simulink model "hw4q1a"  (R2019b)
settings: Solver=FixedStepAuto  StartTime=0.0  StopTime=20  FixedStep=0.01  RelTol=1e-3
libraries: slident x2
settings Model: Creator=axs2437  LastModifiedBy=axs2437
settings DataIOCC: ReturnWorkspaceOutputs=off

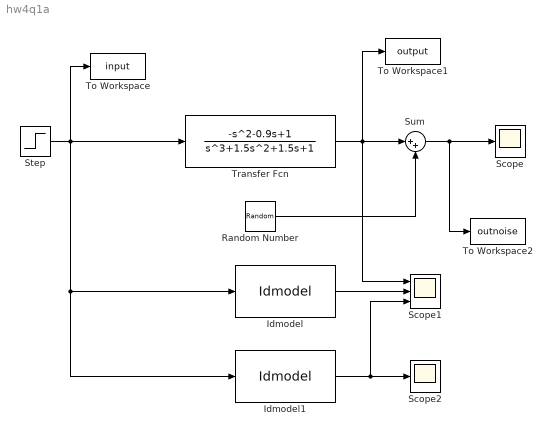
== system hw4q1a ==
  Idmodel : slident/Models/Idmodel  sys=arx321  IC=0  noi=off  seed=[]
      settings: SourceProductName=System Identification Toolbox  SourceProductBaseCode=ID
  Idmodel1 : slident/Models/Idmodel  sys=arx541  IC=0  noi=off  seed=[]
      settings: SourceProductName=System Identification Toolbox  SourceProductBaseCode=ID
  Random Number : RandomNumber  Variance=0.001  SampleTime=0.01
  Scope : Scope
  Scope1 : Scope  NumInputPorts=3
  Scope2 : Scope
  Step : Step  SampleTime=0.01
  Sum : Sum  Inputs=|++
  To Workspace : ToWorkspace  VariableName=input  SampleTime=-1
  To Workspace1 : ToWorkspace  VariableName=output  SampleTime=-1
  To Workspace2 : ToWorkspace  VariableName=outnoise  SampleTime=-1
  Transfer Fcn : TransferFcn  Numerator=[-1 -0.9 1]  Denominator=[1 1.5 1.5 1]
  wires:
  Step/1 -> Idmodel1/1, Idmodel/1, Transfer Fcn/1, To Workspace/1
  Transfer Fcn/1 -> Sum/1, Scope1/1, To Workspace1/1
  Random Number/1 -> Sum/2
  Sum/1 -> To Workspace2/1, Scope/1
  Idmodel/1 -> Scope1/2
  Idmodel1/1 -> Scope2/1, Scope1/3
